simulink model "rlwatertank_simulation_model6"  (R2020b)
settings: Solver=ode45  StartTime=0.0  StopTime=inf  RelTol=1e-3  EnableMultiTasking=on
undefined symbols (not defined in the file): DiscIntNeverNeededParam
libraries: simulink x4, rllib x1
settings Model: Creator=The MathWorks, Inc.  LastModifiedBy=Ferdy
settings DataIOCC: LimitDataPoints=on  SaveFormat=Array  ReturnWorkspaceOutputs=off  SignalLoggingName=logsOut
settings OptimizationCC: ExpressionDepthLimit=2147483647  InitFltsAndDblsToZero=on  LifeSpan=inf
settings DebuggingCC: SaveWithParameterizedLinksMsg=none  UnderspecifiedInitializationDetection=Classic  MergeDetectMultiDrivingBlocksExec=none  SignalResolutionControl=TryResolveAllWithWarning  MultiTaskDSMMsg=warning  FcnCallInpInsideContextMsg=warning  AllowSymbolicDim=off  StateNameClashWarn=warning  SFUnexpectedBacktrackingDiag=warning  SFNoUnconditionalDefaultTransitionDiag=warning  SFExecutionAtInitializationDiag=none  ArithmeticOperatorsInVariantConditions=warning
settings HardwareCC: ProdBitPerPointer=32  ProdBitPerSizeT=32  ProdBitPerPtrDiffT=32  ProdLargestAtomicFloat=None  ProdIntDivRoundTo=Undefined  ProdEndianess=Unspecified  ProdWordSize=32  ProdHWDeviceType=Specified
settings ModelReferenceCC: PropagateSignalLabelsOutOfModel=off
settings SFSimCC: SimUseLocalCustomCode=off  CustomCodeUndefinedFunction=UseInterfaceOnly
settings RTWCC: RTWUseLocalCustomCode=off
settings CodeAppCC: StateflowObjectComments=on
settings GRTTargetCC: TargetFcnLib=ansi_tfl_tmw.mat  TargetLangStandard=C89/C90 (ANSI)  CombineOutputUpdateFcns=off  GRTInterface=on
settings ConfigComp: CovMetricSettings=dw  CovSaveCumulativeToWorkspaceVar=on  CovSaveSingleToWorkspaceVar=on  CovExternalEMLEnable=off

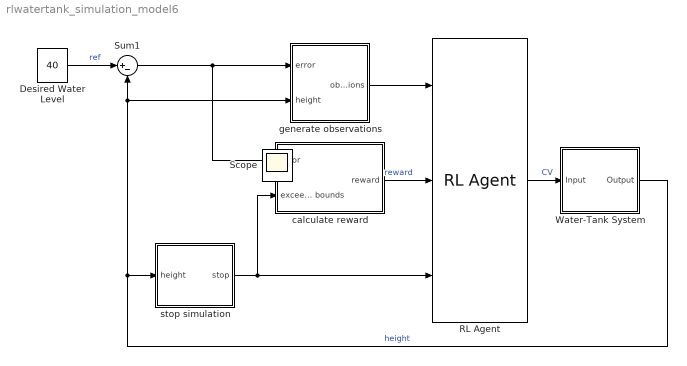
== system rlwatertank_simulation_model6 ==
  Desired Water Level : Constant  Value=40
  RL Agent : rllib/RL Agent  Agent=agent  ProvideReward=on  ProvideIsDone=on  ProvideCumRwd=off  TreatAsDirectFeedthrough=on  CollectLoggedSignals=on  CollectModelStates=on
      settings: SourceProductName=Reinforcement Learning
  Sum1 : Sum  Inputs=|+-  SaturateOnIntegerOverflow=on
  Water-Tank System : Subsystem
  calculate reward : Subsystem
  generate observations : Subsystem
  stop simulation : Subsystem
  Scope : Scope
  wires:
  Desired Water Level/1 -> Sum1/1  "ref"
  Sum1/1 -> calculate reward/1(error), generate observations/1(error)
  Water-Tank System/1(Output) -> stop simulation/1(height), generate observations/2(height), Sum1/2  "height"
  RL Agent/1 -> Water-Tank System/1(Input)  "CV"
  stop simulation/1(stop) -> RL Agent/3, calculate reward/2(exceeds bounds)
  calculate reward/1(reward) -> RL Agent/2  "reward"
  generate observations/1(observations) -> RL Agent/1

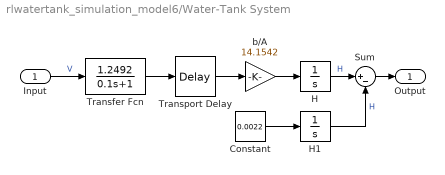
== system rlwatertank_simulation_model6/Water-Tank System ==
  Input : Inport
  Constant : Constant  Value=0.0022
  H : Integrator
  H1 : Integrator
  Sum : Sum  Inputs=|+-
  Transfer Fcn : TransferFcn  Numerator=[1.2492]  Denominator=[0.1 1]
  Transport Delay : TransportDelay  DelayTime=0.09
  b/A : Gain  Gain=14.1542  SaturateOnIntegerOverflow=on  OutDataTypeStr=Inherit: Same as input  ParamDataTypeStr=Inherit: Same as input
  Output : Outport  VectorParamsAs1DForOutWhenUnconnected=off
  wires:
  Input/1 -> Transfer Fcn/1  "V"
  Transfer Fcn/1 -> Transport Delay/1
  Transport Delay/1 -> b/A/1
  b/A/1 -> H/1
  Constant/1 -> H1/1
  H/1 -> Sum/1  "H"
  Sum/1 -> Output/1
  H1/1 -> Sum/2  "H"

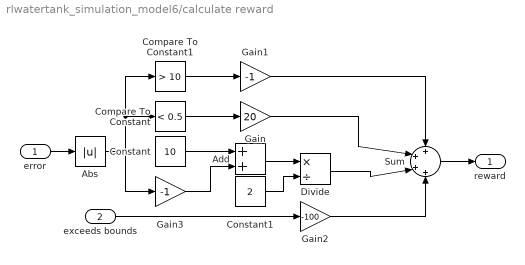
== system rlwatertank_simulation_model6/calculate reward ==
  error : Inport
  exceeds bounds : Inport  Port=2
  Abs : Abs
  Add : Sum
  Compare To Constant : simulink/Logic and Bit Operations/Compare To Constant  relop=<  const=0.5  OutDataTypeStr=boolean
  Compare To Constant1 : simulink/Logic and Bit Operations/Compare To Constant  relop=>  const=10  OutDataTypeStr=boolean
  Constant : Constant  Value=10
  Constant1 : Constant  Value=2
  Divide : Product  Inputs=*/
  Gain : Gain  Gain=20
  Gain1 : Gain  Gain=-1
  Gain2 : Gain  Gain=-100
  Gain3 : Gain  Gain=-1
  Sum : Sum  Inputs=++++  OutDataTypeStr=double
  reward : Outport  VectorParamsAs1DForOutWhenUnconnected=off
  wires:
  Gain2/1 -> Sum/4
  Gain/1 -> Sum/2
  Compare To Constant/1 -> Gain/1
  Sum/1 -> reward/1
  exceeds bounds/1 -> Gain2/1
  error/1 -> Abs/1
  Abs/1 -> Gain3/1, Compare To Constant1/1, Compare To Constant/1
  Compare To Constant1/1 -> Gain1/1
  Gain1/1 -> Sum/1
  Constant/1 -> Add/1
  Gain3/1 -> Add/2
  Add/1 -> Divide/1
  Constant1/1 -> Divide/2
  Divide/1 -> Sum/3

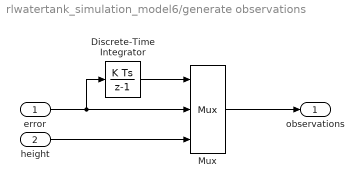
== system rlwatertank_simulation_model6/generate observations ==
  error : Inport
  height : Inport  Port=2
  Discrete-Time Integrator : DiscreteIntegrator  ICPrevOutput=DiscIntNeverNeededParam  ICPrevScaledInput=DiscIntNeverNeededParam
  Mux : Mux  Inputs=3
  observations : Outport  VectorParamsAs1DForOutWhenUnconnected=off
  wires:
  height/1 -> Mux/3
  Discrete-Time Integrator/1 -> Mux/1
  error/1 -> Discrete-Time Integrator/1, Mux/2
  Mux/1 -> observations/1

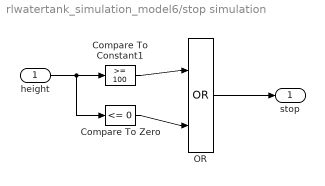
== system rlwatertank_simulation_model6/stop simulation ==
  height : Inport
  Compare To Constant1 : simulink/Logic and Bit Operations/Compare To Constant  relop=>=  const=100  OutDataTypeStr=boolean
  Compare To Zero : simulink/Logic and Bit Operations/Compare To Zero  relop=<=  OutDataTypeStr=boolean
  OR : Logic  Operator=OR  IconShape=distinctive  AllPortsSameDT=off  OutDataTypeStr=boolean
  stop : Outport  VectorParamsAs1DForOutWhenUnconnected=off
  wires:
  height/1 -> Compare To Zero/1, Compare To Constant1/1
  Compare To Zero/1 -> OR/2
  Compare To Constant1/1 -> OR/1
  OR/1 -> stop/1
